simulink library "SimscapeCustomComponents_lib"  (R2025b)
settings: Solver=VariableStepAuto  StartTime=0.0  StopTime=10.0  RelTol=1e-3
undefined symbols (not defined in the file or in its folder): base, baseVdc, capacity, DiscIntNeverNeededParam, ee_sli_rtmsupport, filterInductance, freqeuncy, frequency, gcbh, gflInverter, gfmInverter, iMaxPU, Inertia, initialSOC, plantRating, solar, Ts, ups, Vac, windSystem, windTurbine
libraries: fl_lib x397, nesl_utility x171, eeGeneralControl x85, ee_lib x82, simulink x72, datacenter_lib x68, eeTransforms x38, slpidlib x24, buildingEnergy_lib x20, SimscapeFluids_lib x17, eeSinusoidalMeasurementV2 x8, eePwmGenerator x8
(part 3 of 24)

== system SimscapeCustomComponents_lib/Microgrid and Renewables/Sources ==
  Generator Integrated : Subsystem  Variant=on  VariantControlMode=label  LabelModeActiveChoice=Detailed  mask(Generator){fidelity=Detailed, genRating=5700, Vac=6600, frequency=50, polePairs=1, pu_speed_reference=1, droop_percentage=1, pu_load_reference_setpoint=1, T_G=0.01, T_CH=0.001, base_torque=18000, pu_torque0=18000}
      mask prompts: fidelity "Modeling Option"; genRating "Generator Rating (kW)"; Vac "Rated AC side voltage (phase-phase RMS) (V)"; frequency "Rated electrical frequency at AC side (Hz)"; polePairs "Number of pole pairs"; pu_speed_reference "Speed reference, (pu)"; droop_percentage "Percentage droop, (%)"; pu_load_reference_setpoint "Load reference setpoint, (pu)"; T_G "Time constant of governor, (s)"; T_CH "Time constant of main inlet volumes and steam chest, (s)"; base_torque "Base torque, (N*m)"; pu_torque0 "Initial torque, (pu)"
      mask help:
      | This block models a Generator. The detailed variant models AVR, Exciter, Prime mover, and Governer. The simplified variant is based on load torque and a constant field circuit current. Select simplified mode for faster simulation using fixed efficiency and rated power.
      |
      | Provide load reference as input
      settings: CopyFcn=set_param(gcbh,'LinkStatus','none');
      mask Help: web('Generator.html')
      mask TypeOptions fidelity: Detailed | Simplified
      mask Callback fidelity:
      | detailedTabs = {'generatorDetailed','exciterParam','governerParam',};
      |     simplifiedTabs = {'generatorSimplified'};
      |     component.mask.fidelitySelection(detailedTabs,simplifiedTabs);
      |     component.mask.fidelitySelection;
      mask TypeOptions pu_speed_reference:
      | Detailed/Governor and
      | Prime Mover
      | /pu_speed_reference
      mask TypeOptions droop_percentage:
      | Detailed/Governor and
      | Prime Mover
      | /droop_percentage
      mask TypeOptions pu_load_reference_setpoint:
      | Detailed/Governor and
      | Prime Mover
      | /pu_load_reference_setpoint
      mask TypeOptions T_G:
      | Detailed/Governor and
      | Prime Mover
      | /T_G
      mask TypeOptions T_CH:
      | Detailed/Governor and
      | Prime Mover
      | /T_CH
      mask TypeOptions base_torque:
      | Detailed/Governor and
      | Prime Mover
      | /base_torque
      mask TypeOptions pu_torque0:
      | Detailed/Governor and
      | Prime Mover
      | /pu_torque0
      mask DialogControl generalDetailed Prompt: General
      mask DialogControl editMachine Prompt: Edit machine parameters
      mask DialogControl editMachine Callback:
      | blockFidelity = get_param(gcb,'fidelity');
      |     blockPath = [gcb,'/',blockFidelity,'/','Machine'];
      |     component.mask.openBlock(blockPath);
      mask DialogControl editInertia Prompt: Edit inertia parameters
      mask DialogControl editInertia Callback:
      | blockPath = [gcb,'/','Detailed','/','Inertia'];
      |     component.mask.openBlock(blockPath);
      mask DialogControl exciterParam Prompt: Exciter
      mask DialogControl fieldParam Prompt: Edit field circuit parameters
      mask DialogControl fieldParam Callback:
      | blockPath = [gcb,'/','Detailed','/','AVR and Exciter','/','Exciter'];
      |     component.mask.openBlock(blockPath);
      mask DialogControl avrParam Prompt: Edit AVR parameters
      mask DialogControl avrParam Callback:
      | blockPath = [gcb,'/','Detailed','/','AVR and Exciter','/','AVR'];
      |     component.mask.openBlock(blockPath);
      mask DialogControl governerParam Prompt: Governer and Prime Mover
  Solar Plant : Subsystem  InitFcn=%solar.mask.restoreSolarLink(gcb);  mask(Solar Plant){capDC=0.4, converterFidelity=Average, fSw=20, ratedVoltage=690, nSeries=30, nParallel=536}
      mask prompts: capDC "DC bus capacitance (F)"; converterFidelity "Converter Fidelity"; fSw "Switching Frequency (kHz)"; ratedVoltage "Rated voltage on AC side (V)"; nSeries "Number of panels in series"; nParallel "Number of panels in parallel"
      mask help: This block represents the physical interface between the solar panels and the power converter. It models the electrical and dynamic characteristics of the solar panels connected to a converter, while expecting an external control signal for operation
      settings: CopyFcn=set_param(gcbh,'LinkStatus','none');  PreSaveFcn=%solar.mask.restoreSolarLink(gcb);  CloseFcn=%solar.mask.restoreSolarLink(gcb);
      mask TypeOptions converterFidelity: Converter/converterFidelity
      mask Callback converterFidelity: component.mask.converterFidelityPlant;
      mask TypeOptions fSw: Converter/fSw
      mask DialogControl Container4 Prompt: General
      mask DialogControl editSolarCell Prompt: Edit Solar Cell Parameters
      mask DialogControl editSolarCell Callback:
      | blockPath = [gcb,'/','PV Array'];
      | component.mask.openBlock(blockPath);;
      mask DialogControl editConverter Prompt: Edit converter parameters
      mask DialogControl editConverter Callback:
      | converterFidelity = get_param(gcb,'converterFidelity');
      | blockPath = [gcb,'/','Converter','/',converterFidelity,'/','Converter'];
      | component.mask.openBlock(blockPath);
      mask Display: image('solar_plant.png');
  Solar Plant Integrated : Subsystem  Variant=on  VariantControlMode=label  LabelModeActiveChoice=Simplified  mask(Solar){fidelity=Simplified, plantRating=480e3, Vac=690, frequency=50, iMaxPU=1.2, efficiency=100, baseVoltageDC=1500, nParallel=536, nSeries=30, capacitance=0.04, filterInductance=1e-5, filterResistance=1e-3, panelType=Poly-crystalline, panelRating=48, Isc=9.36, Voc=38.6, irradianceSTC=1000, temperatureSTC=290, alpha=0.005, beta=-0.005, mode=Maximum power point tracking, converterFidelity=Switching, fSw=20}
      mask prompts: fidelity "Modeling Option"; plantRating "Solar Plant Rating (kW)"; Vac "Rated AC side voltage (phase-phase RMS) (V)"; frequency "Rated electrical frequency at AC side (Hz)"; iMaxPU "Maximum converter current (pu)"; efficiency "Converter Efficiency (%)"; baseVoltageDC "Voltage on DC side (V)"; nParallel "Number of panels in parallel"; nSeries "Number of panels in series"; capacitance "DC bus capacitance (F)"; filterInductance "Filter inductance (H)"; filterResistance "Filter series resistance (Ohm)"; panelType "Panel Type"; panelRating "Panel Rating (W)"; Isc "Short-circuit current (A)"; Voc "Open-circuit voltage (V)"; irradianceSTC "Irradiance at STC (W/m² )"; temperatureSTC "Temperature at STC (°K)"; alpha "Temperature co-efficient for current (A/°K)"; beta "Temperature co-efficient for voltage (V/°K)"; mode "Operating Mode"; converterFidelity "Converter Fidelity"; fSw "Switching Frequency (kHz)"
      mask help: This block models a Solar PV plant. The detailed variant models MPPT, voltage and current controllers. The simplified variant is based on Anderson's translational equations. Select simplified mode for faster simulation using fixed efficiency and rated power.
      settings: CopyFcn=set_param(gcbh,'LinkStatus','none');
      mask Help: web('SolarPlant.html')
      mask TypeOptions fidelity: Detailed | Simplified
      mask Callback fidelity: component.mask.fidelitySelection;
      mask TypeOptions nParallel: Detailed/PV Plant & Controller/PV Plant/nParallel
      mask TypeOptions nSeries: Detailed/PV Plant & Controller/PV Plant/nSeries
      mask TypeOptions panelType: Poly-crystalline | Mono-crystalline | Cadmium-Telluride | Others
      mask Callback panelType: component.mask.selectSolarPanelType;
      mask TypeOptions mode: Maximum power point tracking | Power reference
      mask Callback mode:
      | % choice = get_param(gcb,'mode');
      | % blockPath = [gcb,'/','Solar','/','Simplified','/','Solar_Plant'];
      | % blockHandle = get_param(blockPath, 'Handle');
      | % if strcmp(choice,'Maximum power point tracking')
      | %     set_param(blockPath,'modelling_option','ModellingOption.maximumPower');
      | % else
      | %     set_param(blockPath,'modelling_option','ModellingOption.powerReference');
      | % end
      mask TypeOptions converterFidelity: Detailed/PV Plant & Controller/PV Plant/converterFidelity
      mask Callback converterFidelity: component.mask.setSwitchingFrequency;
      mask TypeOptions fSw: Detailed/PV Plant & Controller/PV Plant/fSw
      mask DialogControl generalDetailed Prompt: General
      mask DialogControl cellDetailed Prompt: Solar Cell
      mask DialogControl partsCatalog Prompt: Click to choose from parts catalog
      mask DialogControl partsCatalog Callback: component.mask.openParamManager;
      mask DialogControl panelCalculation Prompt: Calculate number of panels
      mask DialogControl panelCalculation Callback: component.mask.setPanelNumber;
      mask DialogControl configureSolarCell Prompt: Edit Solar Cell Parameters
      mask DialogControl configureSolarCell Callback:
      | blockPath = [gcb,'/','Detailed','/','PV Plant & Controller','/','PV Plant','/','PV Array'];
      |     component.mask.openBlock(blockPath);
      mask DialogControl controllerDetailed Prompt: Solar PV Controller
      mask DialogControl configurePVController Prompt: Edit MPPT Controller
      mask DialogControl configurePVController Callback:
      | blockPath = [gcb,'/','Detailed','/','PV Plant & Controller','/','Controller','/','MPPT','/','Solar PV Controller'];
      |     component.mask.openBlock(blockPath);
      mask DialogControl configurePRefControl Prompt: Edit Power Reference Controller
      mask DialogControl configurePRefControl Callback:
      | blockPath = [gcb,'/','Detailed','/','PV Plant & Controller','/','Controller','/','Power Reference','/','Power Reference Controller'];
      |     component.mask.openBlock(blockPath);
      mask DialogControl cellSimplified Prompt: Solar Cell
      mask DialogControl converter Prompt: Converter
      mask DialogControl editConverter Prompt: Edit converter parameters
      mask DialogControl editConverter Callback:
      | converterFidelity = get_param(gcb,'converterFidelity');
      | blockPath = [gcb,'/','Detailed','/','PV Plant & Controller','/','PV Plant','/','Converter','/',converterFidelity,'/','Converter'];
      | component.mask.openBlock(blockPath);
      mask Display: image('solarPlant.png');
  Wind Plant : Subsystem  mask(Wind Plant){ratedVoltage=690, Vdc=0, capDC=0.4, airDensity=1.225, turbineRadius=83, pitch=1, TSR=1, cp=1, wt=0.01, rt=0.01, p=2, psim=1, Rs=0.1, Ld=0.01, Lq=0.01, converterFidelity=Average, fSw=0}
      mask prompts: ratedVoltage "Rated voltage on AC side (V)"; Vdc "DC bus voltage (V)"; capDC "DC bus capacitance (F)"; airDensity "Air density (kg/m^3)"; turbineRadius "Turbine radius (m)"; pitch "Pitch angle vector (deg)"; TSR "Tip speed ratio"; cp "Power coefficient table, Cp(beta,TSR)"; wt "Wind velocity threshold (m/s)"; rt "Rotational velocity threshold (rad/s)"; p "Number of pole pairs"; psim "PMSM flux linkage (Wb)"; Rs "Stator resistance (Ohm)"; Ld "Stator d-axis inductance (H)"; Lq "Stator q-axis inductance (H)"; converterFidelity "Converter Fidelity"; fSw "Switching Frequency (kHz)"
      mask help: This block represents the physical interface between the wind turbine and the power converters. It models the electrical and dynamic characteristics of the wind turbine connected to a converter, while expecting an external control signal for operation
      settings: CopyFcn=set_param(gcbh,'LinkStatus','none');
      mask TypeOptions capDC: Back-to-Back Converters/capDC
      mask TypeOptions converterFidelity: Back-to-Back Converters/converterFidelity
      mask Callback converterFidelity: component.mask.setSwitchingFrequency;
      mask TypeOptions fSw: Back-to-Back Converters/fSw
      mask DialogControl Container4 Prompt: General
      mask DialogControl Container5 Prompt: Wind Turbine
      mask DialogControl editWindTurbine Prompt: Edit Wind Turbine Parameters
      mask DialogControl editWindTurbine Callback:
      | blockPath = [gcb,'/','Wind Turbine'];
      | component.mask.openBlock(blockPath);
      mask DialogControl Container6 Prompt: PMSG
      mask DialogControl editMachine Prompt: Edit PMSG Parameters
      mask DialogControl editMachine Callback:
      | blockPath = [gcb,'/','PMSG'];
      | component.mask.openBlock(blockPath);
      mask DialogControl Container7 Prompt: Converter
      mask DialogControl editMSConverter Prompt: Edit machine side converter parameters
      mask DialogControl editMSConverter Callback:
      | converterFidelity = get_param(gcb,'converterFidelity');
      | if strcmp(converterFidelity,'Average')
      |     blockPath = [gcb,'/','Back-to-Back Converters','/',converterFidelity,'/','Machine Side Converter'];
      | else
      |     blockPath = [gcb,'/','Back-to-Back Converters','/',converterFidelity,'/','Machine Side Converter','/','Converter'];
      | end
      | component.mask.openBlock(blockPath);
      mask DialogControl editGSConverter Prompt: Edit grid side converter parameters
      mask DialogControl editGSConverter Callback:
      | converterFidelity = get_param(gcb,'converterFidelity');
      | if strcmp(converterFidelity,'Average')
      |     blockPath = [gcb,'/','Back-to-Back Converters','/',converterFidelity,'/','Grid Side Converter'];
      | else
      |     blockPath = [gcb,'/','Back-to-Back Converters','/',converterFidelity,'/','Grid Side Converter','/','Converter'];
      | end
      | component.mask.openBlock(blockPath);
      mask Display: image('windFarmPlant.png');
  Wind Plant Integrated : Subsystem  Variant=on  VariantControlMode=label  LabelModeActiveChoice=Detailed  mask(Wind){fidelity=Detailed, plantRating=1.6e3, Vac=690, frequency=50, iMaxPU=1.2, efficiency=100, baseVoltageDC=1500, airDensity=1.225, turbineRadius=83, pitch=1, TSR=1, cp=1, wt=0.01, rt=0.01, p=1, psim=10, Rs=0.1, Ld=0.001, Lq=0.001, capacitance=0.04, filterInductance=1e-5, filterResistance=1e-3, converterFidelity=Switching, fSw=20}
      mask prompts: fidelity "Modeling Option"; plantRating "Wind Farm Rating (kW)"; Vac "Rated AC side voltage (phase-phase RMS) (V)"; frequency "Rated electrical frequency at AC side (Hz)"; iMaxPU "Maximum converter current (pu)"; efficiency "Converter Efficiency (%)"; baseVoltageDC "Voltage on DC side (V)"; airDensity "Air density (kg/m^3)"; turbineRadius "Turbine radius (m)"; pitch "Pitch angle vector (deg)"; TSR "Tip speed ratio"; cp "Power coefficient table, Cp(beta,TSR)"; wt "Wind velocity threshold (m/s)"; rt "Rotational velocity threshold (rad/s)"; p "Number of pole pairs"; psim "PMSM flux linkage (Wb)"; Rs "Stator resistance (Ohm)"; Ld "Stator d-axis inductance (H)"; Lq "Stator q-axis inductance (H)"; capacitance "DC bus capacitance (F)"; filterInductance "Filter inductance (H)"; filterResistance "Filter series resistance (Ohm)"; converterFidelity "Converter Fidelity"; fSw "Switching Frequency (kHz)"
      mask help: This block models a detailed Type -4 ind farm with the MPPT Controller. The wind farm comprises a permanent magnnet synhronous machine connected to the main grid via back-to-back converters. Select simplified mode for faster simulation using fixed efficiency and rated power.
      settings: CopyFcn=set_param(gcbh,'LinkStatus','none');
      mask Help: web('WIndFarm.html')
      mask TypeOptions fidelity: Detailed | Simplified
      mask Callback fidelity:
      | detailedTabs = {'windDetailed','controllerDetailed','converter'};
      |     simplifiedTabs = {'windSimplified'};
      |     component.mask.fidelitySelection(detailedTabs,simplifiedTabs);
      mask TypeOptions airDensity: Detailed/Wind System/airDensity
      mask TypeOptions turbineRadius: Detailed/Wind System/turbineRadius
      mask TypeOptions pitch: Detailed/Wind System/pitch
      mask TypeOptions TSR: Detailed/Wind System/TSR
      mask TypeOptions cp: Detailed/Wind System/cp
      mask TypeOptions wt: Detailed/Wind System/wt
      mask TypeOptions rt: Detailed/Wind System/rt
      mask TypeOptions p: Detailed/Wind System/p
      mask TypeOptions psim: Detailed/Wind System/psim
      mask TypeOptions Rs: Detailed/Wind System/Rs
      mask TypeOptions Ld: Detailed/Wind System/Ld
      mask TypeOptions Lq: Detailed/Wind System/Lq
      mask TypeOptions converterFidelity: Detailed/Wind Turbine and Converters/Wind Plant/converterFidelity
      mask Callback converterFidelity:
      | converterFidelity = get_param(gcb,'converterFidelity');
      | blockPath = [gcb,'/','Detailed','/','Wind Turbine and Converters','/','Wind Plant','/','Back-to-Back Converters'];
      | % if strcmp(converterFidelity,'Average')
      | %     blockPath = [gcb,'/','Detailed','/','Wind Turbine and Converters','/','Wind Plant','/','Back-to-Back Converters'];
      | % else
      | %     blockPath = [gcb,'/','Detailed','/','Wind Turbine and Converters','/','Wind Plant','/','Back-to-Back Converters'];
      | % end
      | component.mask.converterFidelity(blockPath)
      mask TypeOptions fSw: Detailed/Wind Turbine and Converters/Wind Plant/fSw
      mask DialogControl generalDetailed Prompt: General
      mask DialogControl windDetailed Prompt: Wind Turbine
      mask DialogControl configureWindTurbine Prompt: Edit wind turbine parameters
      mask DialogControl configureWindTurbine Callback:
      | blockPath = [gcb,'/','Detailed','/','Wind Turbine and Converters','/','Wind Plant','/','Wind Turbine'];
      |     component.mask.openBlock(blockPath);
      mask DialogControl Container10 Prompt: PMSM
      mask DialogControl configurePMSM Prompt: Edit PMSM parameters
      mask DialogControl configurePMSM Callback:
      | blockPath = [gcb,'/','Detailed','/','Wind Turbine and Converters','/','Wind Plant','/','PMSG'];
      |  component.mask.openBlock(blockPath);
      mask DialogControl controllerDetailed Prompt: Controller
      mask DialogControl configureWindController Prompt: Edit Wind Controller
      mask DialogControl configureWindController Callback:
      | blockPath = [gcb,'/','Detailed','/','Wind Turbine and Converters','/','Wind Controller'];
      |     component.mask.openBlock(blockPath);
      mask DialogControl windSimplified Prompt: Wind Turbine
      mask DialogControl editWindFarm Prompt: Edit wind farm
      mask DialogControl editWindFarm Callback:
      | blockPath = [gcb,'/','Simplified','/','Wind farm'];
      | component.mask.openBlock(blockPath);
      mask DialogControl converter Prompt: Converter
      mask DialogControl editMSConverter Prompt: Edit machine side converter parameters
      mask DialogControl editMSConverter Callback:
      | blockFidelity = get_param(gcb,'fidelity');
      | converterFidelity = get_param(gcb,'converterFidelity');
      | if strcmp(converterFidelity,'Average')
      |     blockPath = [gcb,'/',blockFidelity,'/','Wind Turbine and Converters','/','Wind Plant','/','Back-to-Back Converters','/',converterFidelity,'/','Machine Side Converter'];
      | else
      |     blockPath = [gcb,'/',blockFidelity,'/','Wind Turbine and Converters','/','Wind Plant','/','Back-to-Back Converters','/',converterFidelity,'/','Machine Side Converter','/','Converter'];
      | end
      | component.mask.openBlock(blockPath);
      mask DialogControl editGSConverter Prompt: Edit grid side converter parameters
      mask DialogControl editGSConverter Callback:
      | blockFidelity = get_param(gcb,'fidelity');
      | converterFidelity = get_param(gcb,'converterFidelity');
      | if strcmp(converterFidelity,'Average')
      |     blockPath = [gcb,'/',blockFidelity,'/','Wind Turbine and Converters','/','Wind Plant','/','Back-to-Back Converters','/',converterFidelity,'/','Grid Side Converter'];
      | else
      |     blockPath = [gcb,'/',blockFidelity,'/','Wind Turbine and Converters','/','Wind Plant','/','Back-to-Back Converters','/',converterFidelity,'/','Grid Side Converter','/','Converter'];
      | end
      | component.mask.openBlock(blockPath);
      mask Display: image('wind_plant.png');
  solar_plant : microgridRenewables_lib/solar_plant  port_option=ee.enum.threePhasePort.composite  FRated=60 Hz  VRated=415 V  PlantRating=100e3 W  modelling_option=ModellingOption.maximumPower  Vdc=1000 V  IMaxPU=1.2  efficiency=100  IrRef=100 W/m^2  T=298 K  PVTech=PanelTechnology.polycrystallinePanel  PanelRating=100 W  VocRef=100 V  IscRef=100 A  alpha=0.005 1/K  beta=-0.005 1/K  delta=0.111
      settings: InternalSimscapePortConfiguration="{\"Bottom\":[],\"Left\":[{\"id\":\"Ir\",\"label\":\"Ir\",\"type\":\"input\"},{\"id\":\"Tsim\",\"label\":\"T\",\"type\":\"input\"}],\"Right\":[{\"id\":\"N\",\"label\":\"~\",\"type\":\"foundation.electrical.three_phase\"},{\"id\":\"l\",\"label\":\"l\",\"type\":\"output\"},{\"id\":\"p\",\"label\":\"p\",\"type\":\"output\"}],\"Top\":[]}"
  wind_farm : microgridRenewables_lib/wind_farm  port_option=ee.enum.threePhasePort.composite  FRated=60 Hz  VRated=415 V  IMaxPU=1.2  PlantRating=100e3 W  modelling_option=ModellingOption.maximumPower  airDensity=1.225 kg/m^3  powercoefficient_option=PowerCoefficient.tableLookUp  TurbineRating=100 W  turbineBlades=3  turbineRadius=1 m  efficiency=100  vWindRated=22 m/s  cutInSpeed=3 m/s  cutOffSpeed=22 m/s  pitch_TLU=[0, 3, 5, 10, 20, 90] deg  lambda_TLU=[0, 2, 4, 6, 8, 10, 12, 14, 15]  Cp_TLU=[0.0010, 0.0161, 0.1446, 0.3865, 0.5009, 0.4404, 0.2545, 0.0002, -0.1384; 0.0016, 0.0173, 0.1079, 0.2676, 0.3779, 0.4111, 0.3838, 0.3176, 0.2753; 0.0027, 0.0197, 0.1151, 0.2606, 0.3469, 0.3558, 0.3069, 0.2222, 0.1718; 0.0054, 0.0283, 0.1315, 0.2364, 0.2589, 0.2022, 0.0929, -0.0455, -0.1204; 0.0109, 0.0536, 0.1320, 0.1256, 0.0120, -0.1752, -0.4017, -0.6435, -0.7655; -0.01 * ones(1, 9)]
      settings: InternalSimscapePortConfiguration="{\"Bottom\":[],\"Left\":[{\"id\":\"vWind\",\"label\":\"V\",\"type\":\"input\"},{\"id\":\"pitch\",\"label\":\"β\",\"type\":\"input\"}],\"Right\":[{\"id\":\"N\",\"label\":\"~\",\"type\":\"foundation.electrical.three_phase\"},{\"id\":\"l\",\"label\":\"I\",\"type\":\"output\"},{\"id\":\"p\",\"label\":\"p\",\"type\":\"output\"}],\"Top\":[]}"

== system SimscapeCustomComponents_lib/Microgrid and Renewables/Storage ==
  BESS GFL Simplified : Subsystem  VariantControl=Grid Following  mask(BESS GFL Simplified){plantRating=2.2e3, Vac=690, frequency=50, iMaxPU=1.2, efficiency=100, bessVoltage=1500, maxSOC=0.95, minSOC=0.1}
      mask prompts: plantRating "BESS Rating (kW)"; Vac "Rated AC side voltage (phase-phase RMS) (V)"; frequency "Rated electrical frequency at AC side (Hz)"; iMaxPU "Maximum converter current (pu)"; efficiency "Converter Efficiency (%)"; bessVoltage "Nominal BESS voltage (V)"; maxSOC "Maximum operating SOC"; minSOC "Minimum operating SOC"
      mask help: This block models a BESS that synchronizes with grid voltage and frequency using simplified control representation. This block is designed for computational efficiency, ideal for system-level studies in strong grid conditions where detailed transient behavior is less critical.
      settings: CopyFcn=set_param(gcbh,'LinkStatus','none');
      mask Help: web('BESSGFLSimplified.html')
      mask DialogControl generalDetailed Prompt: General
      mask DialogControl Container5 Prompt: Battery
      mask DialogControl editBattery Prompt: Edit battery parameters
      mask DialogControl editBattery Callback:
      | blockPath = [gcb,'/','Battery'] ;
      | component.mask.openBlock(blockPath);
  BESS GFM Simplified : Subsystem  VariantControl=Grid Forming  mask(BESS GFM Simplified){plantRating=480e3, Vac=690, frequency=50, Vdc=1500, iMaxPU=1.2, efficiency=100, activeDroop=1e-4, reactiveDroop=0.02, initialSOC=initialSOC, maxSOC=0.95, minSOC=0.1, capacityType=Fixed, capacity=capacity}
      mask prompts: plantRating "BESS Rating (kW)"; Vac "Rated AC side voltage (phase-phase RMS) (V)"; frequency "Rated electrical frequency at AC side (Hz)"; Vdc "Nominal DC bus voltage (V)"; iMaxPU "Maximum converter current (pu)"; efficiency "Converter Efficiency (%)"; activeDroop "Active droop"; reactiveDroop "Reactive droop"; initialSOC "Initial SOC"; maxSOC "Maximum operating SOC"; minSOC "Minimum operating SOC"; capacityType "Battery charge capacity"; capacity "Battery capacity (Ah)"
      mask help: This block models a BESS with generating voltage and frequency reference capabilities. It is optimized for faster simulations while maintaining essential grid-forming behavior, making it suitable for large-scale stability studies or planning scenarios where detailed converter dynamics are not required.
      settings: CopyFcn=set_param(gcbh,'LinkStatus','none');
      mask Help: web('BESSGFMSimplified.html')
      mask TypeOptions capacityType: Fixed | Infinite
      mask Callback capacityType: component.mask.configureBatteryCapacity;
      mask DialogControl generalDetailed Prompt: General
      mask DialogControl Container5 Prompt: Battery
  BESS Integrated : Subsystem  Variant=on  VariantControlMode=label  LabelModeActiveChoice=Detailed  mask(Battery Energy Storage System (BESS)){fidelity=Detailed, bessController=Grid Forming, plantRating=480e3, Vac=690, frequency=50, iMaxPU=1.2, efficiency=100, baseVoltageDC=1500, filterInductance=1e-5, filterResistance=1e-3, maxSOC=0.95, minSOC=0.1, converterFidelity=Switching, fSw=20, activeDroop=1e-3, reactiveDroop=1e-3, maxSOCGFM=0.95, minSOCGFM=0.1, initialSOC=0.9, capacityType=Fixed, capacity=0}
      mask prompts: fidelity "Modeling Option"; bessController "Operating Mode"; plantRating "BESS Rating (kW)"; Vac "Rated AC side voltage (phase-phase RMS) (V)"; frequency "Rated electrical frequency at AC side (Hz)"; iMaxPU "Maximum converter current (pu)"; efficiency "Converter Efficiency (%)"; baseVoltageDC "Voltage on DC side (V)"; filterInductance "Filter inductance (H)"; filterResistance "Filter series resistance (Ohm)"; maxSOC "Maximum  operating SOC"; minSOC "Minimum  operating SOC"; converterFidelity "Converter Fidelity"; fSw "Switching Frequency (kHz)"; activeDroop "Active droop"; reactiveDroop "Reactive droop"; maxSOCGFM "Maximum  operating SOC"; minSOCGFM "Minimum  operating SOC"; initialSOC "Initial SOC"; capacityType "Battery charge capacity"; capacity "Battery capacity (Ah)"
      mask help:
      | This block represents a flexible BESS that can be configured for different operational modes and modeling fidelities. It supports Grid-Following (GFL) and Grid-Forming (GFM) control strategies, along with two fidelity levels:
      |
      | Detailed – captures dynamic control loops and converter behavior for accurate transient analysis.
      | Simplified – optimized for faster simulations while preserving essential system characteristics.
      settings: CopyFcn=set_param(gcbh,'LinkStatus','none');
      mask Help: web('BESS.html')
      mask TypeOptions fidelity: Detailed | Simplified
      mask Callback fidelity:
      | component.mask.fidelitySelection;
      |     fidelity = get_param(gcb,'fidelity');
      |     mode = get_param(gcb,'bessController');
      |     maskObj = Simulink.Mask.get(gcb);
      |     allNames = {maskObj.Parameters.Name};
      |     effIdx = find(strcmp(allNames, 'efficiency'));
      |     tabGFL = maskObj.getDialogControl('cellSimplified');
      |     tabGFM = maskObj.getDialogControl('cellSimplifiedGFM');
      |     if strcmp(fidelity,'Simplified')
      |         maskObj.Parameters(effIdx).Visible = 'on';
      |         if strcmp(mode,'Grid Following')
      |             tabGFL.Visible = 'on';
      |             tabGFM.Visible = 'off';
      |         else
      |             tabGFL.Visible = 'off';
      |             tabGFM.Visible = 'on';
      |         end
      |     else
      |         maskObj.Parameters(effIdx).Visible = 'off';
      |         tabGFL.Visible = 'off';
      |         tabGFM.Visible = 'off';
      |     end
      mask TypeOptions bessController: Grid Following | Grid Forming
      mask Callback bessController:
      | fidelity = get_param(gcb,'fidelity');
      | mode = get_param(gcb,'bessController');
      | if strcmp(fidelity,'Detailed')
      |     component.mask.setBESSController;
      | else
      |     blockPath = [gcb,'/','Simplified'];
      |     component.mask.setBESSController(blockPath);
      | end
      | maskObj = Simulink.Mask.get(gcb);
      | tabGFL = maskObj.getDialogControl('cellSimplified');
      | tabGFM = maskObj.getDialogControl('cellSimplifiedGFM');
      | if strcmp(fidelity,'Simplified')
      |     if strcmp(mode,'Grid Following')
      |         tabGFL.Visible = 'on';
      |         tabGFM.Visible = 'off';
      |     else
      |         tabGFL.Visible = 'off';
      |         tabGFM.Visible = 'on';
      |     end
      | else
      |     tabGFL.Visible = 'off';
      |     tabGFM.Visible = 'off';
      | end
      mask TypeOptions converterFidelity: Detailed/BESS Plant/converterFidelity
      mask Callback converterFidelity:
      | blockPath = [gcb,'/','Detailed','/','BESS Plant','/','Converter'];
      | component.mask.converterFidelity(blockPath);
      mask TypeOptions fSw: Detailed/PV Plant & Controller/PV Plant/fSw
      mask TypeOptions initialSOC: Simplified/Grid Forming/initialSOC
      mask TypeOptions capacityType: Simplified/Grid Forming/capacityType
      mask Callback capacityType: component.mask.configureBatteryCapacity;
      mask TypeOptions capacity: Simplified/Grid Forming/capacity
      mask DialogControl generalDetailed Prompt: General
      mask DialogControl cellDetailed Prompt: Battery
      mask DialogControl configureBattery Prompt: Edit battery parameters
      mask DialogControl configureBattery Callback:
      | blockPath = [gcb,'/','Detailed','/','BESS Plant','/','Battery'] ;
      |     component.mask.openBlock(blockPath);
      mask DialogControl controllerDetailed Prompt: BESS Controller
      mask DialogControl configureBESSController Prompt: Edit BESS Controller
      mask DialogControl configureBESSController Callback:
      | controllerType = get_param(gcb,'bessController');
      |     blockPath = [gcb,'/','Detailed','/','BESS Controller','/',controllerType];
      |     component.mask.openBlock(blockPath);
      mask DialogControl cellSimplified Prompt: Battery
      mask DialogControl configureBatterySimplified Prompt: Edit battery parameters
      mask DialogControl configureBatterySimplified Callback:
      | mode = get_param(gcb,'bessController');
      |     blockPath = [gcb,'/','Simplified','/',mode,'/','Battery'] ;
      |     if strcmp(mode,'Grid Following')
      |         component.mask.openBlock(blockPath);
      |     end
      mask DialogControl converter Prompt: Converter
      mask DialogControl editConverter Prompt: Edit converter parameters
      mask DialogControl editConverter Callback:
      | converterFidelity = get_param(gcb,'converterFidelity');
      | blockPath = [gcb,'/','Detailed','/','BESS Plant','/','Converter','/',converterFidelity,'/','Converter'];
      | component.mask.openBlock(blockPath);
      mask DialogControl cellSimplifiedGFM Prompt: Battery
      mask Display: image('battery_detailed.png');
  BESS Plant : Subsystem  mask(BESS Plant){converterFidelity=Average, fSw=20, ratedVoltage=690}
      mask prompts: converterFidelity "Converter Fidelity"; fSw "Switching Frequency (kHz)"; ratedVoltage "Rated voltage on AC side (V)"
      mask help: This block represents the physical interface between the battery and the power converter. It models the electrical and dynamic characteristics of the battery system connected to a converter, while expecting an external control signal for operation
      settings: CopyFcn=set_param(gcbh,'LinkStatus','none');
      mask TypeOptions converterFidelity: Converter/converterFidelity
      mask Callback converterFidelity: component.mask.converterFidelityPlant;
      mask TypeOptions fSw: Converter/fSw
      mask DialogControl Container4 Prompt: General
      mask DialogControl editBattery Prompt: Edit battery parameters
      mask DialogControl editBattery Callback:
      | blockPath = [gcb,'/','Battery'];
      | component.mask.openBlock(blockPath);
      mask DialogControl editConverter Prompt: Edit converter parameters
      mask DialogControl editConverter Callback:
      | converterFidelity = get_param(gcb,'converterFidelity');
      | blockPath = [gcb,'/','Converter','/',converterFidelity,'/','Converter'];
      | component.mask.openBlock(blockPath);
      mask Display: image('battery_1.png');

== system SimscapeCustomComponents_lib/Building Energy Management/Building/Room with Air Volume ==
  Array Connection3 : SimscapeArrayConnection  Domain=foundation.thermal.thermal  NumScalarElements=5
  PS Selector : fl_lib/Physical Signals/Nonlinear Operators/PS Selector  ix=indxS
      settings: InternalSimscapePortConfiguration="{\"Bottom\":[],\"Left\":[{\"id\":\"I\",\"label\":\"\",\"type\":\"input\"}],\"Right\":[{\"id\":\"O\",\"label\":\"\",\"type\":\"output\"}],\"Top\":[]}"
  Room Volume : buildingEnergy_lib/Room Volume  N1=1  N2=5  iniT=iniT K  length=roomLen m  width=roomWid m  height=roomHgt m
      settings: InternalSimscapePortConfiguration="{\"Bottom\":[],\"Left\":[{\"id\":\"S\",\"label\":\"S\",\"type\":\"input\"}],\"Right\":[{\"id\":\"T\",\"label\":\"T\",\"type\":\"output\"}],\"Top\":[{\"id\":\"M1\",\"label\":\"M1\",\"type\":\"foundation.thermal.thermal\"},{\"id\":\"M2\",\"label\":\"M2\",\"type\":\"foundation.thermal.thermal\"}]}"
  ar1 : fl_lib/Thermal/Thermal Elements/Convective Heat Transfer  thermal_type=foundation.enum.constant_variable.constant  area=roomLen*roomWid m^2  heat_tr_coeff=htc W/(K*m^2)  min_heat_tr_coeff=1e-3 W/(K*m^2)  T_specify=off  T_priority=None  T=0 K  T_nominal_specify=off  T_nominal_value=1  T_nominal_unit=K  Q_specify=off  Q_priority=None  Q=0 W  Q_nominal_specify=off  Q_nominal_value=1  Q_nominal_unit=W
  ar2 : fl_lib/Thermal/Thermal Elements/Convective Heat Transfer  thermal_type=foundation.enum.constant_variable.constant  area=roomLen*roomWid m^2  heat_tr_coeff=htc W/(K*m^2)  min_heat_tr_coeff=1e-3 W/(K*m^2)  T_specify=off  T_priority=None  T=0 K  T_nominal_specify=off  T_nominal_value=1  T_nominal_unit=K  Q_specify=off  Q_priority=None  Q=0 W  Q_nominal_specify=off  Q_nominal_value=1  Q_nominal_unit=W
  ar3 : fl_lib/Thermal/Thermal Elements/Convective Heat Transfer  thermal_type=foundation.enum.constant_variable.constant  area=roomHgt*roomWid m^2  heat_tr_coeff=htc W/(K*m^2)  min_heat_tr_coeff=1e-3 W/(K*m^2)  T_specify=off  T_priority=None  T=0 K  T_nominal_specify=off  T_nominal_value=1  T_nominal_unit=K  Q_specify=off  Q_priority=None  Q=0 W  Q_nominal_specify=off  Q_nominal_value=1  Q_nominal_unit=W
  ar4 : fl_lib/Thermal/Thermal Elements/Convective Heat Transfer  thermal_type=foundation.enum.constant_variable.constant  area=roomLen*roomHgt m^2  heat_tr_coeff=htc W/(K*m^2)  min_heat_tr_coeff=1e-3 W/(K*m^2)  T_specify=off  T_priority=None  T=0 K  T_nominal_specify=off  T_nominal_value=1  T_nominal_unit=K  Q_specify=off  Q_priority=None  Q=0 W  Q_nominal_specify=off  Q_nominal_value=1  Q_nominal_unit=W
  ar5 : fl_lib/Thermal/Thermal Elements/Convective Heat Transfer  thermal_type=foundation.enum.constant_variable.constant  area=roomHgt*roomWid m^2  heat_tr_coeff=htc W/(K*m^2)  min_heat_tr_coeff=1e-3 W/(K*m^2)  T_specify=off  T_priority=None  T=0 K  T_nominal_specify=off  T_nominal_value=1  T_nominal_unit=K  Q_specify=off  Q_priority=None  Q=0 W  Q_nominal_specify=off  Q_nominal_value=1  Q_nominal_unit=W
  ar6 : fl_lib/Thermal/Thermal Elements/Convective Heat Transfer  thermal_type=foundation.enum.constant_variable.constant  area=roomLen*roomHgt m^2  heat_tr_coeff=htc W/(K*m^2)  min_heat_tr_coeff=1e-3 W/(K*m^2)  T_specify=off  T_priority=None  T=0 K  T_nominal_specify=off  T_nominal_value=1  T_nominal_unit=K  Q_specify=off  Q_priority=None  Q=0 W  Q_nominal_specify=off  Q_nominal_value=1  Q_nominal_unit=W
  S : PMIOPort  Side=Left
  W4 : PMIOPort  Port=2  Side=Left
  W3 : PMIOPort  Port=3  Side=Left
  W2 : PMIOPort  Port=4  Side=Right
  T : PMIOPort  Port=5  Side=Right
  W1 : PMIOPort  Port=6  Side=Right
  Bottom : PMIOPort  Port=7  Side=Right
  Top : PMIOPort  Port=8  Side=Left
  connections:
  Array Connection3/RConn1 -- Room Volume/LConn3
  Room Volume/RConn1 -- T/RConn1
  ar6/RConn1 -- W1/RConn1
  ar5/RConn1 -- W2/RConn1
  ar4/RConn1 -- W3/RConn1
  ar3/RConn1 -- W4/RConn1
  Top/RConn1 -- ar1/RConn1
  ar2/RConn1 -- Bottom/RConn1
  Array Connection3/LConn1 -- ar2/LConn1
  ar3/LConn1 -- Array Connection3/LConn2
  ar4/LConn1 -- Array Connection3/LConn3
  ar5/LConn1 -- Array Connection3/LConn4
  ar6/LConn1 -- Array Connection3/LConn5
  PS Selector/RConn1 -- Room Volume/LConn1
  S/RConn1 -- PS Selector/LConn1
  Room Volume/LConn2 -- ar1/LConn1

== system SimscapeCustomComponents_lib/Building Energy Management/Building/Room with Radiator ==
  Array Connection3 : SimscapeArrayConnection  Domain=foundation.thermal.thermal  NumScalarElements=6
  PS Selector : fl_lib/Physical Signals/Nonlinear Operators/PS Selector  ix=indxS
      settings: InternalSimscapePortConfiguration="{\"Bottom\":[],\"Left\":[{\"id\":\"I\",\"label\":\"\",\"type\":\"input\"}],\"Right\":[{\"id\":\"O\",\"label\":\"\",\"type\":\"output\"}],\"Top\":[]}"
  PS Selector1 : fl_lib/Physical Signals/Nonlinear Operators/PS Selector  ix=indxV
      settings: InternalSimscapePortConfiguration="{\"Bottom\":[],\"Left\":[{\"id\":\"I\",\"label\":\"\",\"type\":\"input\"}],\"Right\":[{\"id\":\"O\",\"label\":\"\",\"type\":\"output\"}],\"Top\":[]}"
  Room Volume1 : buildingEnergy_lib/Room Volume  N1=1  N2=6  iniT=iniT K  length=roomLen m  width=roomWid m  height=roomHgt m
      settings: InternalSimscapePortConfiguration="{\"Bottom\":[],\"Left\":[{\"id\":\"S\",\"label\":\"S\",\"type\":\"input\"}],\"Right\":[{\"id\":\"T\",\"label\":\"T\",\"type\":\"output\"}],\"Top\":[{\"id\":\"M1\",\"label\":\"M1\",\"type\":\"foundation.thermal.thermal\"},{\"id\":\"M2\",\"label\":\"M2\",\"type\":\"foundation.thermal.thermal\"}]}"
  Room Wall Radiator1 : buildingEnergy_lib/Room Wall Radiator  pipeHydrDia=pipeHydrDiaR m  pipeLength=pipeLenR m  pipeArea=pipeCrossSectionalAreaR m^2  pipeRoughness=pipeRoughnessR m  htc=htc W/(K*m^2)  iniTemperature=iniT K
      settings: InternalSimscapePortConfiguration="{\"Bottom\":[],\"Left\":[{\"id\":\"TL_V\",\"label\":\"V\",\"type\":\"input\"},{\"id\":\"TL_A\",\"label\":\"A\",\"type\":\"foundation.thermal_liquid.thermal_liquid\"}],\"Right\":[{\"id\":\"M\",\"label\":\"R\",\"type\":\"foundation.thermal.thermal\"},{\"id\":\"TL_B\",\"label\":\"B\",\"type\":\"foundation.thermal_liquid.thermal_liquid\"}],\"Top\":[]}"
  ar1 : fl_lib/Thermal/Thermal Elements/Convective Heat Transfer  thermal_type=foundation.enum.constant_variable.constant  area=roomLen*roomWid m^2  heat_tr_coeff=htc W/(K*m^2)  min_heat_tr_coeff=1e-3 W/(K*m^2)  T_specify=off  T_priority=None  T=0 K  T_nominal_specify=off  T_nominal_value=1  T_nominal_unit=K  Q_specify=off  Q_priority=None  Q=0 W  Q_nominal_specify=off  Q_nominal_value=1  Q_nominal_unit=W
  ar2 : fl_lib/Thermal/Thermal Elements/Convective Heat Transfer  thermal_type=foundation.enum.constant_variable.constant  area=roomLen*roomWid m^2  heat_tr_coeff=htc W/(K*m^2)  min_heat_tr_coeff=1e-3 W/(K*m^2)  T_specify=off  T_priority=None  T=0 K  T_nominal_specify=off  T_nominal_value=1  T_nominal_unit=K  Q_specify=off  Q_priority=None  Q=0 W  Q_nominal_specify=off  Q_nominal_value=1  Q_nominal_unit=W
  ar3 : fl_lib/Thermal/Thermal Elements/Convective Heat Transfer  thermal_type=foundation.enum.constant_variable.constant  area=roomHgt*roomWid m^2  heat_tr_coeff=htc W/(K*m^2)  min_heat_tr_coeff=1e-3 W/(K*m^2)  T_specify=off  T_priority=None  T=0 K  T_nominal_specify=off  T_nominal_value=1  T_nominal_unit=K  Q_specify=off  Q_priority=None  Q=0 W  Q_nominal_specify=off  Q_nominal_value=1  Q_nominal_unit=W
  ar4 : fl_lib/Thermal/Thermal Elements/Convective Heat Transfer  thermal_type=foundation.enum.constant_variable.constant  area=roomLen*roomHgt m^2  heat_tr_coeff=htc W/(K*m^2)  min_heat_tr_coeff=1e-3 W/(K*m^2)  T_specify=off  T_priority=None  T=0 K  T_nominal_specify=off  T_nominal_value=1  T_nominal_unit=K  Q_specify=off  Q_priority=None  Q=0 W  Q_nominal_specify=off  Q_nominal_value=1  Q_nominal_unit=W
  ar5 : fl_lib/Thermal/Thermal Elements/Convective Heat Transfer  thermal_type=foundation.enum.constant_variable.constant  area=roomHgt*roomWid m^2  heat_tr_coeff=htc W/(K*m^2)  min_heat_tr_coeff=1e-3 W/(K*m^2)  T_specify=off  T_priority=None  T=0 K  T_nominal_specify=off  T_nominal_value=1  T_nominal_unit=K  Q_specify=off  Q_priority=None  Q=0 W  Q_nominal_specify=off  Q_nominal_value=1  Q_nominal_unit=W
  ar6 : fl_lib/Thermal/Thermal Elements/Convective Heat Transfer  thermal_type=foundation.enum.constant_variable.constant  area=roomLen*roomHgt m^2  heat_tr_coeff=htc W/(K*m^2)  min_heat_tr_coeff=1e-3 W/(K*m^2)  T_specify=off  T_priority=None  T=0 K  T_nominal_specify=off  T_nominal_value=1  T_nominal_unit=K  Q_specify=off  Q_priority=None  Q=0 W  Q_nominal_specify=off  Q_nominal_value=1  Q_nominal_unit=W
  ar7 : fl_lib/Thermal/Thermal Elements/Convective Heat Transfer  thermal_type=foundation.enum.constant_variable.constant  area=pipeLenR*pipeHydrDiaR m^2  heat_tr_coeff=htc W/(K*m^2)  min_heat_tr_coeff=1e-3 W/(K*m^2)  T_specify=off  T_priority=None  T=0 K  T_nominal_specify=off  T_nominal_value=1  T_nominal_unit=K  Q_specify=off  Q_priority=None  Q=0 W  Q_nominal_specify=off  Q_nominal_value=1  Q_nominal_unit=W
  V : PMIOPort  Side=Left
  S : PMIOPort  Port=2  Side=Left
  W4 : PMIOPort  Port=3  Side=Left
  TL_A : PMIOPort  Port=4  Side=Left
  W3 : PMIOPort  Port=5  Side=Left
  TL_B : PMIOPort  Port=6  Side=Right
  W2 : PMIOPort  Port=7  Side=Right
  T : PMIOPort  Port=8  Side=Right
  W1 : PMIOPort  Port=9  Side=Right
  Bottom : PMIOPort  Port=10  Side=Right
  Top : PMIOPort  Port=11  Side=Left
  connections:
  Room Wall Radiator1/RConn2 -- TL_B/RConn1
  Room Volume1/RConn1 -- T/RConn1
  Room Wall Radiator1/LConn2 -- TL_A/RConn1
  ar6/RConn1 -- W1/RConn1
  ar5/RConn1 -- W2/RConn1
  ar4/RConn1 -- W3/RConn1
  ar3/RConn1 -- W4/RConn1
  ar7/RConn1 -- Array Connection3/LConn2
  Top/RConn1 -- ar1/RConn1
  ar2/RConn1 -- Bottom/RConn1
  Array Connection3/LConn3 -- ar3/LConn1
  Array Connection3/LConn4 -- ar4/LConn1
  Array Connection3/LConn5 -- ar5/LConn1
  Array Connection3/LConn6 -- ar6/LConn1
  Room Wall Radiator1/RConn1 -- ar7/LConn1
  ar2/LConn1 -- Array Connection3/LConn1
  Room Wall Radiator1/LConn1 -- PS Selector1/RConn1
  PS Selector1/LConn1 -- V/RConn1
  PS Selector/LConn1 -- S/RConn1
  Room Volume1/LConn1 -- PS Selector/RConn1
  Room Volume1/LConn3 -- Array Connection3/RConn1
  Room Volume1/LConn2 -- ar1/LConn1

== system SimscapeCustomComponents_lib/Building Energy Management/Building/Room with Under-floor Piping ==
  Array Connection3 : SimscapeArrayConnection  Domain=foundation.thermal.thermal  NumScalarElements=5
  PS Selector : fl_lib/Physical Signals/Nonlinear Operators/PS Selector  ix=indxS
      settings: InternalSimscapePortConfiguration="{\"Bottom\":[],\"Left\":[{\"id\":\"I\",\"label\":\"\",\"type\":\"input\"}],\"Right\":[{\"id\":\"O\",\"label\":\"\",\"type\":\"output\"}],\"Top\":[]}"
  PS Selector1 : fl_lib/Physical Signals/Nonlinear Operators/PS Selector  ix=indxV
      settings: InternalSimscapePortConfiguration="{\"Bottom\":[],\"Left\":[{\"id\":\"I\",\"label\":\"\",\"type\":\"input\"}],\"Right\":[{\"id\":\"O\",\"label\":\"\",\"type\":\"output\"}],\"Top\":[]}"
  Room Underfloor Piping : buildingEnergy_lib/Room Underfloor Piping  pipeHydrDia=pipeHydrDiaUFP m  pipeLength=pipeLenUFP m  pipeArea=pipeCrossSectionalAreaUFP m^2  pipeRoughness=pipeRoughnessUFP m  htc=htc W/(K*m^2)  iniTemperature=iniT K
      settings: InternalSimscapePortConfiguration="{\"Bottom\":[],\"Left\":[{\"id\":\"TL_V\",\"label\":\"V\",\"type\":\"input\"},{\"id\":\"TL_A\",\"label\":\"A\",\"type\":\"foundation.thermal_liquid.thermal_liquid\"}],\"Right\":[{\"id\":\"M\",\"label\":\"R\",\"type\":\"foundation.thermal.thermal\"},{\"id\":\"TL_B\",\"label\":\"B\",\"type\":\"foundation.thermal_liquid.thermal_liquid\"}],\"Top\":[]}"
  Room Volume : buildingEnergy_lib/Room Volume  N1=1  N2=5  iniT=iniT K  length=roomLen m  width=roomWid m  height=roomHgt m
      settings: InternalSimscapePortConfiguration="{\"Bottom\":[],\"Left\":[{\"id\":\"S\",\"label\":\"S\",\"type\":\"input\"}],\"Right\":[{\"id\":\"T\",\"label\":\"T\",\"type\":\"output\"}],\"Top\":[{\"id\":\"M1\",\"label\":\"M1\",\"type\":\"foundation.thermal.thermal\"},{\"id\":\"M2\",\"label\":\"M2\",\"type\":\"foundation.thermal.thermal\"}]}"
  Thermal Resistance : fl_lib/Thermal/Thermal Elements/Thermal Resistance  resistance=thermalResFloor K/W  T_specify=off  T_priority=None  T=0 K  T_nominal_specify=off  T_nominal_value=1  T_nominal_unit=K  Q_specify=off  Q_priority=None  Q=0 W  Q_nominal_specify=off  Q_nominal_value=1  Q_nominal_unit=W
  ar1 : fl_lib/Thermal/Thermal Elements/Convective Heat Transfer  thermal_type=foundation.enum.constant_variable.constant  area=roomLen*roomWid m^2  heat_tr_coeff=htc W/(K*m^2)  min_heat_tr_coeff=1e-3 W/(K*m^2)  T_specify=off  T_priority=None  T=0 K  T_nominal_specify=off  T_nominal_value=1  T_nominal_unit=K  Q_specify=off  Q_priority=None  Q=0 W  Q_nominal_specify=off  Q_nominal_value=1  Q_nominal_unit=W
  ar3 : fl_lib/Thermal/Thermal Elements/Convective Heat Transfer  thermal_type=foundation.enum.constant_variable.constant  area=roomHgt*roomWid m^2  heat_tr_coeff=htc W/(K*m^2)  min_heat_tr_coeff=1e-3 W/(K*m^2)  T_specify=off  T_priority=None  T=0 K  T_nominal_specify=off  T_nominal_value=1  T_nominal_unit=K  Q_specify=off  Q_priority=None  Q=0 W  Q_nominal_specify=off  Q_nominal_value=1  Q_nominal_unit=W
  ar4 : fl_lib/Thermal/Thermal Elements/Convective Heat Transfer  thermal_type=foundation.enum.constant_variable.constant  area=roomLen*roomHgt m^2  heat_tr_coeff=htc W/(K*m^2)  min_heat_tr_coeff=1e-3 W/(K*m^2)  T_specify=off  T_priority=None  T=0 K  T_nominal_specify=off  T_nominal_value=1  T_nominal_unit=K  Q_specify=off  Q_priority=None  Q=0 W  Q_nominal_specify=off  Q_nominal_value=1  Q_nominal_unit=W
  ar5 : fl_lib/Thermal/Thermal Elements/Convective Heat Transfer  thermal_type=foundation.enum.constant_variable.constant  area=roomHgt*roomWid m^2  heat_tr_coeff=htc W/(K*m^2)  min_heat_tr_coeff=1e-3 W/(K*m^2)  T_specify=off  T_priority=None  T=0 K  T_nominal_specify=off  T_nominal_value=1  T_nominal_unit=K  Q_specify=off  Q_priority=None  Q=0 W  Q_nominal_specify=off  Q_nominal_value=1  Q_nominal_unit=W
  ar6 : fl_lib/Thermal/Thermal Elements/Convective Heat Transfer  thermal_type=foundation.enum.constant_variable.constant  area=roomLen*roomHgt m^2  heat_tr_coeff=htc W/(K*m^2)  min_heat_tr_coeff=1e-3 W/(K*m^2)  T_specify=off  T_priority=None  T=0 K  T_nominal_specify=off  T_nominal_value=1  T_nominal_unit=K  Q_specify=off  Q_priority=None  Q=0 W  Q_nominal_specify=off  Q_nominal_value=1  Q_nominal_unit=W
  ar8 : fl_lib/Thermal/Thermal Elements/Convective Heat Transfer  thermal_type=foundation.enum.constant_variable.constant  area=pipeLenUFP*pipeHydrDiaUFP/2 m^2  heat_tr_coeff=htc W/(K*m^2)  min_heat_tr_coeff=1e-3 W/(K*m^2)  T_specify=off  T_priority=None  T=0 K  T_nominal_specify=off  T_nominal_value=1  T_nominal_unit=K  Q_specify=off  Q_priority=None  Q=0 W  Q_nominal_specify=off  Q_nominal_value=1  Q_nominal_unit=W
  V : PMIOPort  Side=Left
  S : PMIOPort  Port=2  Side=Left
  W4 : PMIOPort  Port=3  Side=Left
  TL_A : PMIOPort  Port=4  Side=Left
  W3 : PMIOPort  Port=5  Side=Left
  TL_B : PMIOPort  Port=6  Side=Right
  W2 : PMIOPort  Port=7  Side=Right
  T : PMIOPort  Port=8  Side=Right
  W1 : PMIOPort  Port=9  Side=Right
  Bottom : PMIOPort  Port=10  Side=Right
  Top : PMIOPort  Port=11  Side=Left
  connections:
  Room Underfloor Piping/LConn2 -- TL_A/RConn1
  Room Underfloor Piping/RConn2 -- TL_B/RConn1
  Room Volume/RConn1 -- T/RConn1
  ar6/RConn1 -- W1/RConn1
  ar5/RConn1 -- W2/RConn1
  ar4/RConn1 -- W3/RConn1
  ar3/RConn1 -- W4/RConn1
  Thermal Resistance/LConn1 -- Room Underfloor Piping/RConn1 -- ar8/LConn1
  Top/RConn1 -- ar1/RConn1
  Thermal Resistance/RConn1 -- Bottom/RConn1
  ar8/RConn1 -- Array Connection3/LConn1
  Array Connection3/LConn2 -- ar3/LConn1
  ar4/LConn1 -- Array Connection3/LConn3
  ar5/LConn1 -- Array Connection3/LConn4
  ar6/LConn1 -- Array Connection3/LConn5
  PS Selector/LConn1 -- S/RConn1
  Room Underfloor Piping/LConn1 -- PS Selector1/RConn1
  PS Selector1/LConn1 -- V/RConn1
  PS Selector/RConn1 -- Room Volume/LConn1
  Room Volume/LConn3 -- Array Connection3/RConn1
  Room Volume/LConn2 -- ar1/LConn1
